simulink model "problem8"  (R2020b)
settings: Solver=FixedStepDiscrete  StartTime=0.0  StopTime=inf  FixedStep=0.1  RelTol=1e-3  EnableMultiTasking=on
settings Model: ModifiedByFormat=Markus Hornauer  Creator=Markus Hornauer  LastModifiedBy=Markus Hornauer
settings DataIOCC: LimitDataPoints=on  SaveFormat=Array  SignalLoggingSaveFormat=ModelDataLogs  ReturnWorkspaceOutputs=off
settings OptimizationCC: ExpressionDepthLimit=2147483647  LifeSpan=inf
settings DebuggingCC: UnderspecifiedInitializationDetection=Classic  MergeDetectMultiDrivingBlocksExec=none  SolverPrmCheckMsg=warning  FcnCallInpInsideContextMsg=warning  StateNameClashWarn=warning  SFUnexpectedBacktrackingDiag=warning  SFNoUnconditionalDefaultTransitionDiag=warning  SFExecutionAtInitializationDiag=none  ArithmeticOperatorsInVariantConditions=warning
settings HardwareCC: ProdBitPerPointer=32  ProdBitPerSizeT=32  ProdBitPerPtrDiffT=32  ProdLargestAtomicFloat=None  ProdIntDivRoundTo=Undefined  ProdEndianess=Unspecified  ProdWordSize=32  ProdHWDeviceType=32-bit Generic
settings ModelReferenceCC: PropagateSignalLabelsOutOfModel=off
settings SFSimCC: SimUseLocalCustomCode=off  CustomCodeUndefinedFunction=UseInterfaceOnly
settings RTWCC: RTWUseLocalCustomCode=off
settings CodeAppCC: StateflowObjectComments=on
settings GRTTargetCC: TargetLangStandard=C89/C90 (ANSI)  CombineOutputUpdateFcns=off  GRTInterface=on
settings ConfigComp: CovMetricSettings=dw  CovSaveCumulativeToWorkspaceVar=on  CovSaveSingleToWorkspaceVar=on  CovExternalEMLEnable=off  CovSFcnEnable=off

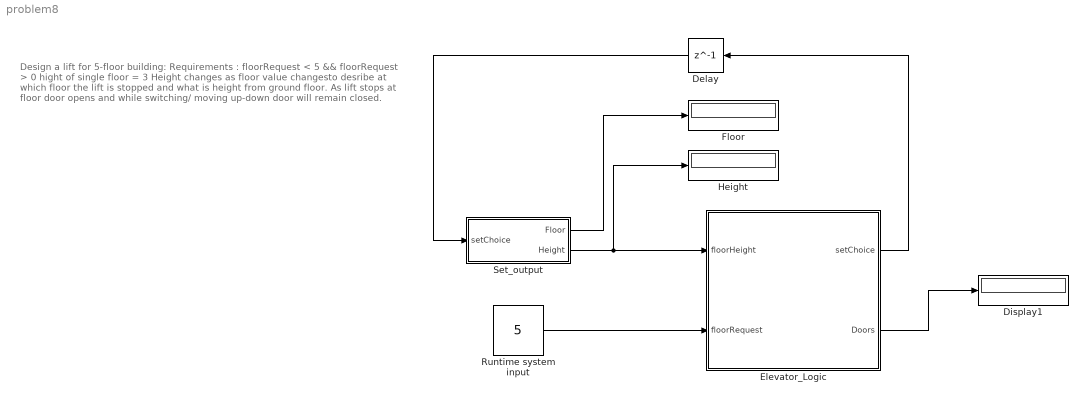
== system problem8 ==
  note: Design a lift for 5-floor building:
      |
      | Requirements :
      | floorRequest < 5 && floorRequest > 0
      |
      | hight of single floor = 3
      |
      | Height changes as floor value changesto desribe at which floor the lift is stopped and what is height from ground floor.
      |
      | As lift stops at floor door opens and while switching/ moving up-down door will remain closed.
  Delay : Delay  DelayLength=1  InitialCondition=3
  Display1 : Display
  Elevator_Logic : Stateflow chart  TreatAsAtomicUnit=on
  Floor : Display
  Height : Display
  Runtime system input : Constant  Value=5
  Set_output : Subsystem  TreatAsAtomicUnit=on
  wires:
  Set_output/2(Height) -> Elevator_Logic/1(floorHeight), Height/1
  Elevator_Logic/1(setChoice) -> Delay/1
  Delay/1 -> Set_output/1(setChoice)
  Elevator_Logic/2(Doors) -> Display1/1
  Runtime system input/1 -> Elevator_Logic/2(floorRequest)
  Set_output/1(Floor) -> Floor/1

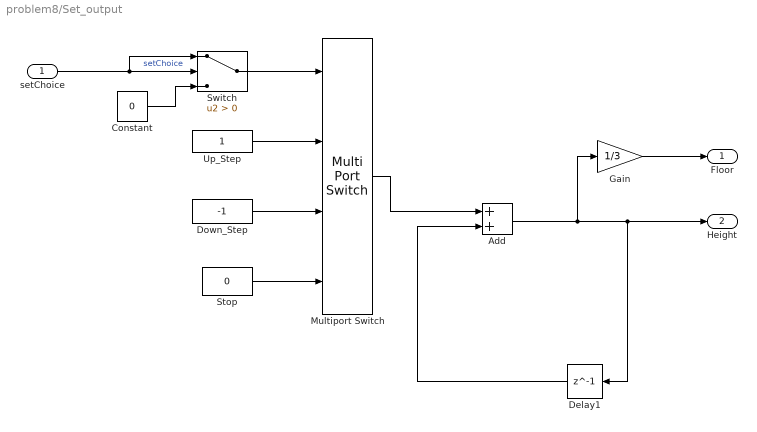
== system problem8/Set_output ==
  setChoice : Inport
  Add : Sum
  Constant : Constant  Value=0
  Delay1 : Delay  DelayLength=1
  Down_Step : Constant  Value=-1
  Gain : Gain  Gain=1/3  OutDataTypeStr=int8
  Multiport Switch : MultiPortSwitch  DiagnosticForDefault=None
  Stop : Constant  Value=0
  Switch : Switch  Criteria=u2 > Threshold
  Up_Step : Constant
  Floor : Outport
  Height : Outport  Port=2
  wires:
  Down_Step/1 -> Multiport Switch/3
  Up_Step/1 -> Multiport Switch/2
  Stop/1 -> Multiport Switch/4
  Multiport Switch/1 -> Add/1
  Add/1 -> Height/1, Delay1/1, Gain/1
  Delay1/1 -> Add/2
  Gain/1 -> Floor/1
  setChoice/1 -> Switch/2, Switch/1  "setChoice"
  Switch/1 -> Multiport Switch/1
  Constant/1 -> Switch/3

== stateflow chart problem8/Elevator_Logic ==
  state Move
    state Entry
    state GoDown
      entry: setChoice = 2;
      Doors = false;
    state Initial_State
      entry: setChoice = 3;
      Doors = false;
    state Stop
      entry: setChoice = 3;
      Doors = true;
    state GoUp
      entry: setChoice = 1;
      Doors = false;
    (default) -> Entry
    Entry -> Initial_State : [result == 1]
    Initial_State -> GoDown [order 3] : [floorHeight > floorRequest * 3]
    GoDown -> Stop : [floorHeight <= floorRequest * 3]
    Stop -> GoDown [order 2] : [floorHeight > floorRequest * 3 + 1]
    Initial_State -> Stop [order 1] : [floorHeight == floorRequest * 3]
    Initial_State -> GoUp [order 2] : [floorHeight < floorRequest * 3]
    Stop -> GoUp [order 1] : [floorHeight < floorRequest * 3 - 1]
    GoUp -> Stop : [floorHeight >= floorRequest * 3]
  state Start
    state state1Check
      en:
    state stateActive
      exit:
      result = 0;
    state StateStop
      entry:
      setChoice = 0;
      during:
      result = CheckReq(floorRequest);
    (default) -> state1Check : {result = CheckReq(floorRequest);}
    state1Check -> stateActive [order 1] : [result == 1]
    state1Check -> StateStop [order 2] : [result == 0]
    StateStop -> state1Check : [hasChanged(floorRequest) || result == 1]
  note: %If given floor request is greater than 5 then lift will not go to that requested floor but stays at same position. And if floor request is less than 5 then go to the floor that is requested.
  note: Graphiccal Function to check request input
  state res = CheckReq(Req) [function]
    (default) -> (junction 37)
    (junction 37) -> (junction 38) [order 1] : [Req > 5]
    (junction 37) -> (junction 39) [order 2] : {res = 1;}
    (junction 38) -> (junction 40) : {res = 0;}
    (junction 40) -> (junction 39)
    (junction 39) -> (junction 41)
  note: %As per the floor request the lift moves from up and down. The value of height is also updated as lift goes up and down.
      | Lift Door is only open when lift is stopped.
  (default) -> Start
  Move -> Start : [hasChanged(floorRequest)]
  Start -> Move : [result == 1]
  data: res function_output double; Req function_input double; setChoice output double; Doors output boolean size=1 =false; result local double; floorHeight input; floorRequest input
